simulink model "GA"  (R2020a)
settings: Solver=VariableStepAuto  StartTime=0.0  StopTime=1  RelTol=1e-3
values from neighbouring files (symbols this model uses):
  b = 0.1    [matlab.mat]
  g = 9.8    [matlab.mat]
  I = 0.006    [matlab.mat]
  l = 0.3    [matlab.mat]
  m = 0.2    [matlab.mat]
  M = 0.5    [matlab.mat]
  q = 0.0132    [matlab.mat]
undefined symbols (not defined in the file or in its folder): k
libraries: simulink x1
settings Model: Creator=akshit  LastModifiedBy=akshit

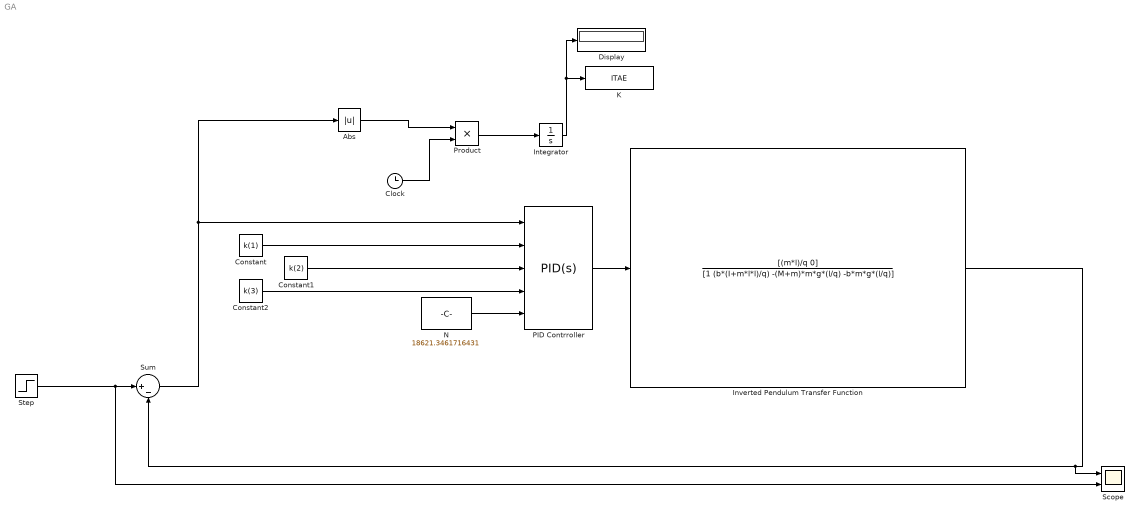
== system GA ==
  Abs : Abs
  Clock : Clock
  Constant : Constant  Value=k(1)
  Constant1 : Constant  Value=k(2)
  Constant2 : Constant  Value=k(3)
  Display : Display
  Integrator : Integrator
  Inverted Pendulum Transfer Function : TransferFcn  Numerator=[(m*l)/q 0]  Denominator=[1 (b*(I+m*l*l)/q) -(M+m)*m*g*(l/q) -b*m*g*(l/q)]
  K : ToWorkspace  VariableName=ITAE  SampleTime=-1
  N : Constant  Value=18621.3461716431
  PID Contrroller : simulink/Continuous/PID Controller  Controller=PID  Form=Parallel  TimeDomain=Continuous-time  UseExternalTs=off  SampleTime=-1  IntegratorMethod=Forward Euler  FilterMethod=Forward Euler  ControllerParametersSource=external  P=1  I=1  D=1  UseFilter=on  N=18621.3461716431  TunerSelectOption=Transfer Function Based (PID Tuner App)  InitialConditionSource=internal  InitialConditionForIntegrator=0  InitialConditionForFilter=0  DifferentiatorICPrevScaledInput=0  ExternalReset=none  TrackingMode=off  Kt=1  LimitOutput=off  UpperSaturationLimit=inf  LowerSaturationLimit=-inf  LinearizeAsGain=on  AntiWindupMode=none  Kb=1  POutMin=[]  POutMax=[]  IOutMin=[]  IOutMax=[]  DOutMin=[]  DOutMax=[]  NOutMin=[]  NOutMax=[]  SumOutMin=[]  SumOutMax=[]  SaturationOutMin=[]  SaturationOutMax=[]  PParamMin=[]  PParamMax=[]  IParamMin=[]  IParamMax=[]  DParamMin=[]  DParamMax=[]  NParamMin=[]  NParamMax=[]  KbParamMin=[]  KbParamMax=[]  KtParamMin=[]  KtParamMax=[]  KbOutMin=[]  KbOutMax=[]  KtOutMin=[]  KtOutMax=[]  IntegratorOutMin=[]  IntegratorOutMax=[]  FilterOutMin=[]  FilterOutMax=[]  SumI1OutMin=[]  SumI1OutMax=[]  SumI2OutMin=[]  SumI2OutMax=[]  SumI3OutMin=[]  SumI3OutMax=[]  SumI4OutMin=[]  SumI4OutMax=[]  SumDOutMin=[]  SumDOutMax=[]  DifferentiatorOutMin=[]  DifferentiatorOutMax=[]  FilterDiffOutCoefMin=[]  FilterDiffOutCoefMax=[]  ReciprocalOutMin=[]  ReciprocalOutMax=[]  SumDenOutMin=[]  SumDenOutMax=[]  SumNumOutMin=[]  SumNumOutMax=[]  DivideOutMin=[]  DivideOutMax=[]  UdiffTsProdOutMin=[]  UdiffTsProdOutMax=[]  NTsProdOutMin=[]  NTsProdOutMax=[]  UintegralTsProdOutMin=[]  UintegralTsProdOutMax=[]  UngainTsProdOutMin=[]  UngainTsProdOutMax=[]  IntegratorContinuousStateAttributes=''  IntegratorStateMustResolveToSignalObject=off  IntegratorRTWStateStorageClass=Auto  FilterContinuousStateAttributes=''  FilterStateMustResolveToSignalObject=off  FilterRTWStateStorageClass=Auto  ParallelPVariant=ExternalParameters  IdealPVariant=Disabled  IVariant=ExternalParameters  DVariant=ExternalParameters  IntegratorVariant=Continuous  SatVariant=Disabled  AWVariant=Passthrough  PCopyVariant=Disabled  TRVariant=Disabled  FdbkBlocksVariant=Forward  IdealPFdbkVariant=Disabled  SatFdbkVariant=Disabled  DerivativeFilterVariant=ContFilter  NVariant=ExternalParameters  NCopyVariant=Disabled  FilterICVariant=InternalICsFilter  IntegratorICVariant=InternalICs  ExternalResetVariant=Disabled  TRSumVariant=Passthrough  SumFdbkVariant=Disabled  SumVariant=Sum_PID  TsampFilterVariant=InternalTs  TsampNgainVariant=Passthrough  TsampIntegralVariant=Passthrough
  Product : Product
  Scope : Scope  NumInputPorts=2
  Step : Step  Time=0.2  SampleTime=0
  Sum : Sum  Inputs=|+-
  wires:
  Inverted Pendulum Transfer Function/1 -> Sum/2, Scope/1
  Sum/1 -> Abs/1, PID Contrroller/1
  PID Contrroller/1 -> Inverted Pendulum Transfer Function/1
  N/1 -> PID Contrroller/5
  Constant/1 -> PID Contrroller/2
  Constant1/1 -> PID Contrroller/3
  Product/1 -> Integrator/1
  Clock/1 -> Product/2
  Abs/1 -> Product/1
  Integrator/1 -> Display/1, K/1
  Constant2/1 -> PID Contrroller/4
  Step/1 -> Scope/2, Sum/1
